simulink model "Chaine_de_conversion_eolienne_25kw"  (R2024a)
settings: Solver=FixedStepAuto  StartTime=0.0  StopTime=10  FixedStep=Ts  RelTol=1e-3
undefined symbols (not defined in the file): A1, A2, A3, A4, A5, A6, C_dc, f, F, G, J, J_PMSG, ki_id_grid, ki_iq_grid, ki_isd, ki_omega, ki_PLL, ki_Q, ki_vdc, kp_id_grid, kp_iq_grid, kp_isd, kp_omega, kp_PLL, kp_Q, kp_vdc, Kt, Lf, Ls, p, Phi_r, R, Rf, rho, Rs, S, Ts, Vdc_ref
libraries: eeGeneralControl x12, slpidlib x8, spsThreePhaseVIMeasurementLib x3, eeTransforms x3, spsCurrentMeasurementLib x3, spsVoltageMeasurementLib x3, spsUniversalBridgeLib x2, spsPWMGenerator2LevelLib x2, powerlib_extras x2, spsRMSLib x2, spsTHDLib x2, spsThreePhaseSeriesRLCBranchLib x1
(part 2 of 2)

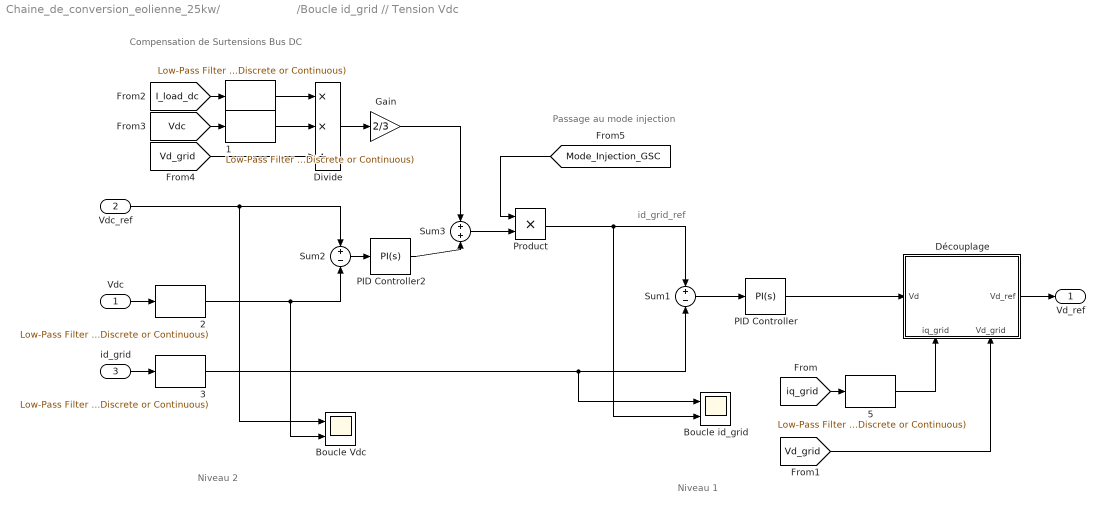
== system Chaine_de_conversion_eolienne_25kw/                       /Boucle id_grid // Tension Vdc ==
  note: Niveau 1
  note: Compensation de Surtensions Bus DC
  note: Passage au mode injection
  note: id_grid_ref
  note: Niveau 2
  Vdc : Inport
  Vdc_ref : Inport  Port=2
  id_grid : Inport  Port=3
  "   " : eeGeneralControl/Low-Pass Filter (Discrete or Continuous)  K=1  T=0.001  B=inf  A=-inf  init_option=Inherited from block input  x0=0  Ts=-1
     {1..3,5} (4 alike) : eeGeneralControl/Low-Pass Filter (Discrete or Continuous)  K=1  T=0.5e-3  B=inf  A=-inf  init_option=Inherited from block input  x0=0  Ts=-1
  Boucle Vdc : Scope  NumInputPorts=2
  "Boucle id_grid   " : Scope  NumInputPorts=2
  Divide : Product  Inputs=**/
  Découplage : Subsystem
      settings: PortSchema="{\"entries\":[{\"content\":{\"sides\":[{\"content\":{\"connectorIds\":[\"In1\"]},\"type\":\"ConnectorPlacement.EquallySpacedRectSide\",\"uuid\":\"7d3af298-2f9f-475a-a651-f5eac2186357\"},{\"content\":{\"connectorIds\":[\"Out1\"],\"side\":\"RIGHT\"},\"type\":\"ConnectorPlacement.EquallySpacedRectSide\",\"uuid\":\"aa22588b-a98c-4a55-adf5-26eaad5d3043\"},{\"content\":{\"side\":\"TOP\"},\"type\":\"ConnectorPlacement.EquallySpacedRectSide\",\"uuid\":\"895af8ff-ad69-460f-8331-727a35d5d5ec\"},{\"content\":{\"connectorIds\":[\"In2\",\"In3\"],\"side\":\"BOTTOM\"},\"type\":\"ConnectorPlacement.EquallySpacedRectSide\",\"uuid\":\"a79db6ec-2ceb-4bca-883f-aa3bf861af08\"}]},\"type\":\"ConnectorPlacement.EquallySpacedConnector\",\"uuid\":\"f85c84fc-5e67-455b-b890-ed27a42cb9c3\"}],\"packageUris\":[\"http://schema.mathworks.com/mf0/Connector/R2020b\"],\"version\":\"1.0\"}"
  Gain : Gain  Gain=2/3
  PID Controller : slpidlib/PID Controller  Controller=PI  Form=Parallel  TimeDomain=Continuous-time  UseExternalTs=off  SampleTime=-1  IntegratorMethod=Forward Euler  FilterMethod=Forward Euler  ControllerParametersSource=internal  P=kp_id_grid  I=ki_id_grid  UseKiTs=off  D=0  UseExternalDerivativeSource=off  N=100  UseFilter=on  TunerSelectOption=Transfer Function Based (PID Tuner App)  InitialConditionSource=internal  InitialConditionForIntegrator=0  InitialConditionForFilter=0  DifferentiatorICPrevScaledInput=0  ExternalReset=none  TrackingMode=off  Kt=1  LimitOutput=off  SatLimitsSource=internal  UpperSaturationLimit=inf  LowerSaturationLimit=-inf  LinearizeAsGain=on  AntiWindupMode=none  Kb=1  LimitIntegrator=off  UpperIntegratorSaturationLimit=inf  LowerIntegratorSaturationLimit=-inf  POutMin=[]  POutMax=[]  IOutMin=[]  IOutMax=[]  DOutMin=[]  DOutMax=[]  NOutMin=[]  NOutMax=[]  SumOutMin=[]  SumOutMax=[]  SaturationOutMin=[]  SaturationOutMax=[]  PParamMin=[]  PParamMax=[]  IParamMin=[]  IParamMax=[]  DParamMin=[]  DParamMax=[]  NParamMin=[]  NParamMax=[]  KbParamMin=[]  KbParamMax=[]  KtParamMin=[]  KtParamMax=[]  KbOutMin=[]  KbOutMax=[]  KtOutMin=[]  KtOutMax=[]  IntegratorOutMin=[]  IntegratorOutMax=[]  FilterOutMin=[]  FilterOutMax=[]  SumI1OutMin=[]  SumI1OutMax=[]  SumI2OutMin=[]  SumI2OutMax=[]  SumI3OutMin=[]  SumI3OutMax=[]  SumI4OutMin=[]  SumI4OutMax=[]  SumDOutMin=[]  SumDOutMax=[]  DifferentiatorOutMin=[]  DifferentiatorOutMax=[]  FilterDiffOutCoefMin=[]  FilterDiffOutCoefMax=[]  ReciprocalOutMin=[]  ReciprocalOutMax=[]  SumDenOutMin=[]  SumDenOutMax=[]  SumNumOutMin=[]  SumNumOutMax=[]  DivideOutMin=[]  DivideOutMax=[]  UdiffTsProdOutMin=[]  UdiffTsProdOutMax=[]  NTsProdOutMin=[]  NTsProdOutMax=[]  UintegralTsProdOutMin=[]  UintegralTsProdOutMax=[]  UngainTsProdOutMin=[]  UngainTsProdOutMax=[]  ClampingZeroOutDataTypeStr=Inherit: Inherit via back propagation  ClampingZeroOutMin=[]  ClampingZeroOutMax=[]  FilterDenConstantOutDataTypeStr=Inherit: Inherit via back propagation  FilterDenConstantOutMin=[]  FilterDenConstantOutMax=[]  PCopyOutDataTypeStr=Inherit: Inherit via back propagation  PCopyOutMin=[]  PCopyOutMax=[]  NCopyOutDataTypeStr=Inherit: Inherit via back propagation  NCopyOutMin=[]  NCopyOutMax=[]  IntegratorContinuousStateAttributes=''  IntegratorStateMustResolveToSignalObject=off  IntegratorRTWStateStorageClass=Auto  FilterContinuousStateAttributes=''  FilterStateMustResolveToSignalObject=off  FilterRTWStateStorageClass=Auto  ParallelPVariant=InternalParameters  IdealPVariant=Disabled  IVariant=InternalParameters  DVariant=Disabled  IntegratorVariant=Continuous  SatVariant=Disabled  AWVariant=Passthrough  PCopyVariant=Disabled  TRVariant=Disabled  FdbkBlocksVariant=Forward  IdealPFdbkVariant=Disabled  SatFdbkVariant=Disabled  DerivativeFilterVariant=Disabled  NVariant=Disabled  NCopyVariant=Disabled_SignalSpec  FilterICVariant=Disabled  IntegratorICVariant=InternalICs  ExternalResetVariant=Disabled  TRSumVariant=Passthrough  SumFdbkVariant=Disabled  SumVariant=Sum_PI  TsampFilterVariant=InternalTs  TsampNgainVariant=Passthrough  TsampIntegralVariant=Disabled_SignalSpec  ExternalSaturationOutDataTypeStr=Inherit: Same as second input  DerivativeSourceVariant=Disabled
  PID Controller2 : slpidlib/PID Controller  Controller=PI  Form=Parallel  TimeDomain=Continuous-time  UseExternalTs=off  SampleTime=-1  IntegratorMethod=Forward Euler  FilterMethod=Forward Euler  ControllerParametersSource=internal  P=kp_vdc  I=ki_vdc  UseKiTs=off  D=0  UseExternalDerivativeSource=off  N=100  UseFilter=on  TunerSelectOption=Transfer Function Based (PID Tuner App)  InitialConditionSource=internal  InitialConditionForIntegrator=0  InitialConditionForFilter=0  DifferentiatorICPrevScaledInput=0  ExternalReset=none  TrackingMode=off  Kt=1  LimitOutput=off  SatLimitsSource=internal  UpperSaturationLimit=inf  LowerSaturationLimit=-inf  LinearizeAsGain=on  AntiWindupMode=none  Kb=1  LimitIntegrator=off  UpperIntegratorSaturationLimit=inf  LowerIntegratorSaturationLimit=-inf  POutMin=[]  POutMax=[]  IOutMin=[]  IOutMax=[]  DOutMin=[]  DOutMax=[]  NOutMin=[]  NOutMax=[]  SumOutMin=[]  SumOutMax=[]  SaturationOutMin=[]  SaturationOutMax=[]  PParamMin=[]  PParamMax=[]  IParamMin=[]  IParamMax=[]  DParamMin=[]  DParamMax=[]  NParamMin=[]  NParamMax=[]  KbParamMin=[]  KbParamMax=[]  KtParamMin=[]  KtParamMax=[]  KbOutMin=[]  KbOutMax=[]  KtOutMin=[]  KtOutMax=[]  IntegratorOutMin=[]  IntegratorOutMax=[]  FilterOutMin=[]  FilterOutMax=[]  SumI1OutMin=[]  SumI1OutMax=[]  SumI2OutMin=[]  SumI2OutMax=[]  SumI3OutMin=[]  SumI3OutMax=[]  SumI4OutMin=[]  SumI4OutMax=[]  SumDOutMin=[]  SumDOutMax=[]  DifferentiatorOutMin=[]  DifferentiatorOutMax=[]  FilterDiffOutCoefMin=[]  FilterDiffOutCoefMax=[]  ReciprocalOutMin=[]  ReciprocalOutMax=[]  SumDenOutMin=[]  SumDenOutMax=[]  SumNumOutMin=[]  SumNumOutMax=[]  DivideOutMin=[]  DivideOutMax=[]  UdiffTsProdOutMin=[]  UdiffTsProdOutMax=[]  NTsProdOutMin=[]  NTsProdOutMax=[]  UintegralTsProdOutMin=[]  UintegralTsProdOutMax=[]  UngainTsProdOutMin=[]  UngainTsProdOutMax=[]  ClampingZeroOutDataTypeStr=Inherit: Inherit via back propagation  ClampingZeroOutMin=[]  ClampingZeroOutMax=[]  FilterDenConstantOutDataTypeStr=Inherit: Inherit via back propagation  FilterDenConstantOutMin=[]  FilterDenConstantOutMax=[]  PCopyOutDataTypeStr=Inherit: Inherit via back propagation  PCopyOutMin=[]  PCopyOutMax=[]  NCopyOutDataTypeStr=Inherit: Inherit via back propagation  NCopyOutMin=[]  NCopyOutMax=[]  IntegratorContinuousStateAttributes=''  IntegratorStateMustResolveToSignalObject=off  IntegratorRTWStateStorageClass=Auto  FilterContinuousStateAttributes=''  FilterStateMustResolveToSignalObject=off  FilterRTWStateStorageClass=Auto  ParallelPVariant=InternalParameters  IdealPVariant=Disabled  IVariant=InternalParameters  DVariant=Disabled  IntegratorVariant=Continuous  SatVariant=Disabled  AWVariant=Passthrough  PCopyVariant=Disabled  TRVariant=Disabled  FdbkBlocksVariant=Forward  IdealPFdbkVariant=Disabled  SatFdbkVariant=Disabled  DerivativeFilterVariant=Disabled  NVariant=Disabled  NCopyVariant=Disabled_SignalSpec  FilterICVariant=Disabled  IntegratorICVariant=InternalICs  ExternalResetVariant=Disabled  TRSumVariant=Passthrough  SumFdbkVariant=Disabled  SumVariant=Sum_PI  TsampFilterVariant=InternalTs  TsampNgainVariant=Passthrough  TsampIntegralVariant=Disabled_SignalSpec  ExternalSaturationOutDataTypeStr=Inherit: Same as second input  DerivativeSourceVariant=Disabled
  Product : Product
  Sum1 : Sum  Inputs=+-
  Sum2 : Sum  Inputs=+-
  Sum3 : Sum
  Vd_ref : Outport
  wires:
  Sum1/1 -> PID Controller/1
  id_grid/1 -> "   3"/1
  Découplage/1(Vd_ref) -> Vd_ref/1
  Sum2/1 -> PID Controller2/1
  Vdc/1 -> "   2"/1
  Vdc_ref/1 -> Boucle Vdc/1, Sum2/1
  Product/1 -> "Boucle id_grid   "/2, Sum1/1
  PID Controller2/1 -> Sum3/2
  PID Controller/1 -> Découplage/1(Vd)
  [iq_grid] -> "   5"/1
  Divide/1 -> Gain/1
  Gain/1 -> Sum3/1
  [Vdc] -> "   1"/1
  [Vd_grid] -> Divide/3
  [I_load_dc] -> "   "/1
  "   "/1 -> Divide/1
  "   1"/1 -> Divide/2
  "   2"/1 -> Boucle Vdc/2, Sum2/2
  "   3"/1 -> Sum1/2, "Boucle id_grid   "/1
  [Vd_grid] -> Découplage/3(Vd_grid)
  "   5"/1 -> Découplage/2(iq_grid)
  Sum3/1 -> Product/2
  [Mode_Injection_GSC] -> Product/1

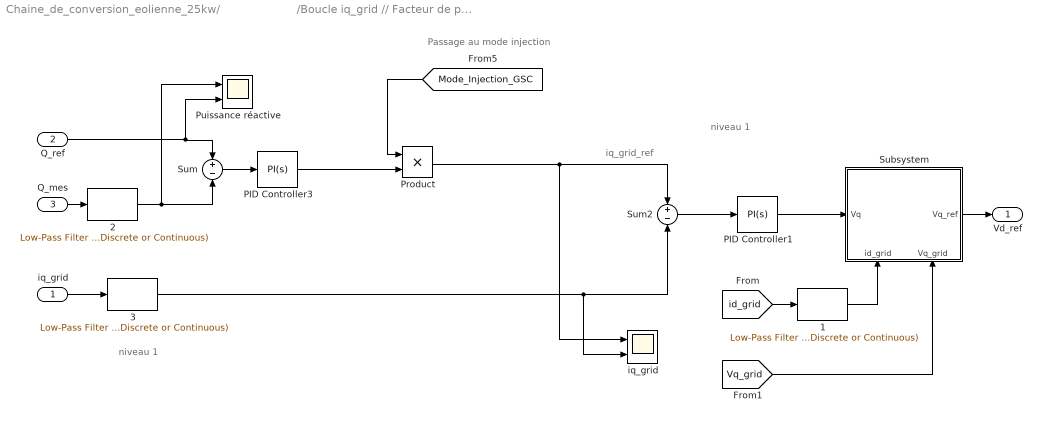
== system Chaine_de_conversion_eolienne_25kw/                       /Boucle iq_grid // Facteur de puissance ==
  note: niveau 1
  note: iq_grid_ref
  note: Passage au mode injection
  note: niveau 1
  iq_grid : Inport
  Q_ref : Inport  Port=2
  Q_mes : Inport  Port=3
  "   1" : eeGeneralControl/Low-Pass Filter (Discrete or Continuous)  K=1  T=0.5e-3  B=inf  A=-inf  init_option=Inherited from block input  x0=0  Ts=-1
  "   2" : eeGeneralControl/Low-Pass Filter (Discrete or Continuous)  K=1  T=0.5e-3  B=inf  A=-inf  init_option=Inherited from block input  x0=0  Ts=-1
  "   3" : eeGeneralControl/Low-Pass Filter (Discrete or Continuous)  K=1  T=0.5e-3  B=inf  A=-inf  init_option=Inherited from block input  x0=0  Ts=-1
  PID Controller1 : slpidlib/PID Controller  Controller=PI  Form=Parallel  TimeDomain=Continuous-time  UseExternalTs=off  SampleTime=-1  IntegratorMethod=Forward Euler  FilterMethod=Forward Euler  ControllerParametersSource=internal  P=kp_iq_grid  I=ki_iq_grid  UseKiTs=off  D=0  UseExternalDerivativeSource=off  N=100  UseFilter=on  TunerSelectOption=Transfer Function Based (PID Tuner App)  InitialConditionSource=internal  InitialConditionForIntegrator=0  InitialConditionForFilter=0  DifferentiatorICPrevScaledInput=0  ExternalReset=none  TrackingMode=off  Kt=1  LimitOutput=off  SatLimitsSource=internal  UpperSaturationLimit=inf  LowerSaturationLimit=-inf  LinearizeAsGain=on  AntiWindupMode=none  Kb=1  LimitIntegrator=off  UpperIntegratorSaturationLimit=inf  LowerIntegratorSaturationLimit=-inf  POutMin=[]  POutMax=[]  IOutMin=[]  IOutMax=[]  DOutMin=[]  DOutMax=[]  NOutMin=[]  NOutMax=[]  SumOutMin=[]  SumOutMax=[]  SaturationOutMin=[]  SaturationOutMax=[]  PParamMin=[]  PParamMax=[]  IParamMin=[]  IParamMax=[]  DParamMin=[]  DParamMax=[]  NParamMin=[]  NParamMax=[]  KbParamMin=[]  KbParamMax=[]  KtParamMin=[]  KtParamMax=[]  KbOutMin=[]  KbOutMax=[]  KtOutMin=[]  KtOutMax=[]  IntegratorOutMin=[]  IntegratorOutMax=[]  FilterOutMin=[]  FilterOutMax=[]  SumI1OutMin=[]  SumI1OutMax=[]  SumI2OutMin=[]  SumI2OutMax=[]  SumI3OutMin=[]  SumI3OutMax=[]  SumI4OutMin=[]  SumI4OutMax=[]  SumDOutMin=[]  SumDOutMax=[]  DifferentiatorOutMin=[]  DifferentiatorOutMax=[]  FilterDiffOutCoefMin=[]  FilterDiffOutCoefMax=[]  ReciprocalOutMin=[]  ReciprocalOutMax=[]  SumDenOutMin=[]  SumDenOutMax=[]  SumNumOutMin=[]  SumNumOutMax=[]  DivideOutMin=[]  DivideOutMax=[]  UdiffTsProdOutMin=[]  UdiffTsProdOutMax=[]  NTsProdOutMin=[]  NTsProdOutMax=[]  UintegralTsProdOutMin=[]  UintegralTsProdOutMax=[]  UngainTsProdOutMin=[]  UngainTsProdOutMax=[]  ClampingZeroOutDataTypeStr=Inherit: Inherit via back propagation  ClampingZeroOutMin=[]  ClampingZeroOutMax=[]  FilterDenConstantOutDataTypeStr=Inherit: Inherit via back propagation  FilterDenConstantOutMin=[]  FilterDenConstantOutMax=[]  PCopyOutDataTypeStr=Inherit: Inherit via back propagation  PCopyOutMin=[]  PCopyOutMax=[]  NCopyOutDataTypeStr=Inherit: Inherit via back propagation  NCopyOutMin=[]  NCopyOutMax=[]  IntegratorContinuousStateAttributes=''  IntegratorStateMustResolveToSignalObject=off  IntegratorRTWStateStorageClass=Auto  FilterContinuousStateAttributes=''  FilterStateMustResolveToSignalObject=off  FilterRTWStateStorageClass=Auto  ParallelPVariant=InternalParameters  IdealPVariant=Disabled  IVariant=InternalParameters  DVariant=Disabled  IntegratorVariant=Continuous  SatVariant=Disabled  AWVariant=Passthrough  PCopyVariant=Disabled  TRVariant=Disabled  FdbkBlocksVariant=Forward  IdealPFdbkVariant=Disabled  SatFdbkVariant=Disabled  DerivativeFilterVariant=Disabled  NVariant=Disabled  NCopyVariant=Disabled_SignalSpec  FilterICVariant=Disabled  IntegratorICVariant=InternalICs  ExternalResetVariant=Disabled  TRSumVariant=Passthrough  SumFdbkVariant=Disabled  SumVariant=Sum_PI  TsampFilterVariant=InternalTs  TsampNgainVariant=Passthrough  TsampIntegralVariant=Disabled_SignalSpec  ExternalSaturationOutDataTypeStr=Inherit: Same as second input  DerivativeSourceVariant=Disabled
  PID Controller3 : slpidlib/PID Controller  Controller=PI  Form=Parallel  TimeDomain=Continuous-time  UseExternalTs=off  SampleTime=-1  IntegratorMethod=Forward Euler  FilterMethod=Forward Euler  ControllerParametersSource=internal  P=kp_Q  I=ki_Q  UseKiTs=off  D=0  UseExternalDerivativeSource=off  N=100  UseFilter=on  TunerSelectOption=Transfer Function Based (PID Tuner App)  InitialConditionSource=internal  InitialConditionForIntegrator=0  InitialConditionForFilter=0  DifferentiatorICPrevScaledInput=0  ExternalReset=none  TrackingMode=off  Kt=1  LimitOutput=off  SatLimitsSource=internal  UpperSaturationLimit=inf  LowerSaturationLimit=-inf  LinearizeAsGain=on  AntiWindupMode=none  Kb=1  LimitIntegrator=off  UpperIntegratorSaturationLimit=inf  LowerIntegratorSaturationLimit=-inf  POutMin=[]  POutMax=[]  IOutMin=[]  IOutMax=[]  DOutMin=[]  DOutMax=[]  NOutMin=[]  NOutMax=[]  SumOutMin=[]  SumOutMax=[]  SaturationOutMin=[]  SaturationOutMax=[]  PParamMin=[]  PParamMax=[]  IParamMin=[]  IParamMax=[]  DParamMin=[]  DParamMax=[]  NParamMin=[]  NParamMax=[]  KbParamMin=[]  KbParamMax=[]  KtParamMin=[]  KtParamMax=[]  KbOutMin=[]  KbOutMax=[]  KtOutMin=[]  KtOutMax=[]  IntegratorOutMin=[]  IntegratorOutMax=[]  FilterOutMin=[]  FilterOutMax=[]  SumI1OutMin=[]  SumI1OutMax=[]  SumI2OutMin=[]  SumI2OutMax=[]  SumI3OutMin=[]  SumI3OutMax=[]  SumI4OutMin=[]  SumI4OutMax=[]  SumDOutMin=[]  SumDOutMax=[]  DifferentiatorOutMin=[]  DifferentiatorOutMax=[]  FilterDiffOutCoefMin=[]  FilterDiffOutCoefMax=[]  ReciprocalOutMin=[]  ReciprocalOutMax=[]  SumDenOutMin=[]  SumDenOutMax=[]  SumNumOutMin=[]  SumNumOutMax=[]  DivideOutMin=[]  DivideOutMax=[]  UdiffTsProdOutMin=[]  UdiffTsProdOutMax=[]  NTsProdOutMin=[]  NTsProdOutMax=[]  UintegralTsProdOutMin=[]  UintegralTsProdOutMax=[]  UngainTsProdOutMin=[]  UngainTsProdOutMax=[]  ClampingZeroOutDataTypeStr=Inherit: Inherit via back propagation  ClampingZeroOutMin=[]  ClampingZeroOutMax=[]  FilterDenConstantOutDataTypeStr=Inherit: Inherit via back propagation  FilterDenConstantOutMin=[]  FilterDenConstantOutMax=[]  PCopyOutDataTypeStr=Inherit: Inherit via back propagation  PCopyOutMin=[]  PCopyOutMax=[]  NCopyOutDataTypeStr=Inherit: Inherit via back propagation  NCopyOutMin=[]  NCopyOutMax=[]  IntegratorContinuousStateAttributes=''  IntegratorStateMustResolveToSignalObject=off  IntegratorRTWStateStorageClass=Auto  FilterContinuousStateAttributes=''  FilterStateMustResolveToSignalObject=off  FilterRTWStateStorageClass=Auto  ParallelPVariant=InternalParameters  IdealPVariant=Disabled  IVariant=InternalParameters  DVariant=Disabled  IntegratorVariant=Continuous  SatVariant=Disabled  AWVariant=Passthrough  PCopyVariant=Disabled  TRVariant=Disabled  FdbkBlocksVariant=Forward  IdealPFdbkVariant=Disabled  SatFdbkVariant=Disabled  DerivativeFilterVariant=Disabled  NVariant=Disabled  NCopyVariant=Disabled_SignalSpec  FilterICVariant=Disabled  IntegratorICVariant=InternalICs  ExternalResetVariant=Disabled  TRSumVariant=Passthrough  SumFdbkVariant=Disabled  SumVariant=Sum_PI  TsampFilterVariant=InternalTs  TsampNgainVariant=Passthrough  TsampIntegralVariant=Disabled_SignalSpec  ExternalSaturationOutDataTypeStr=Inherit: Same as second input  DerivativeSourceVariant=Disabled
  Product : Product
  Puissance réactive : Scope  NumInputPorts=2
  Subsystem : Subsystem
      settings: PortSchema="{\"entries\":[{\"content\":{\"sides\":[{\"content\":{\"connectorIds\":[\"In1\"]},\"type\":\"ConnectorPlacement.EquallySpacedRectSide\",\"uuid\":\"7d3af298-2f9f-475a-a651-f5eac2186357\"},{\"content\":{\"connectorIds\":[\"Out1\"],\"side\":\"RIGHT\"},\"type\":\"ConnectorPlacement.EquallySpacedRectSide\",\"uuid\":\"aa22588b-a98c-4a55-adf5-26eaad5d3043\"},{\"content\":{\"side\":\"TOP\"},\"type\":\"ConnectorPlacement.EquallySpacedRectSide\",\"uuid\":\"895af8ff-ad69-460f-8331-727a35d5d5ec\"},{\"content\":{\"connectorIds\":[\"In2\",\"In3\"],\"side\":\"BOTTOM\"},\"type\":\"ConnectorPlacement.EquallySpacedRectSide\",\"uuid\":\"a79db6ec-2ceb-4bca-883f-aa3bf861af08\"}]},\"type\":\"ConnectorPlacement.EquallySpacedConnector\",\"uuid\":\"f85c84fc-5e67-455b-b890-ed27a42cb9c3\"}],\"packageUris\":[\"http://schema.mathworks.com/mf0/Connector/R2020b\"],\"version\":\"1.0\"}"
  Sum : Sum  Inputs=+-
  Sum2 : Sum  Inputs=+-
  "iq_grid " : Scope  NumInputPorts=2
  Vd_ref : Outport
  wires:
  Sum/1 -> PID Controller3/1
  Sum2/1 -> PID Controller1/1
  iq_grid/1 -> "   3"/1
  Q_mes/1 -> "   2"/1
  Product/1 -> "iq_grid "/1, Sum2/1
  [id_grid] -> "   1"/1
  PID Controller1/1 -> Subsystem/1(Vq)
  Subsystem/1(Vq_ref) -> Vd_ref/1
  [Vq_grid] -> Subsystem/3(Vq_grid)
  "   3"/1 -> Sum2/2, "iq_grid "/2
  Q_ref/1 -> Sum/1, Puissance réactive/2
  "   2"/1 -> Sum/2, Puissance réactive/1
  "   1"/1 -> Subsystem/2(id_grid)
  [Mode_Injection_GSC] -> Product/1
  PID Controller3/1 -> Product/2

== system Chaine_de_conversion_eolienne_25kw/                       /Convertisseur Tension// PWM  ==
  abc_ref : Inport
  Divide3 : Product  Inputs=*/
  PWM Generator (2-Level) : spsPWMGenerator2LevelLib/PWM Generator (2-Level)  ModulatorType=Three-phase bridge (6 pulses)  ModulatorMode=Unsynchronized  Fc=Fc  Pc=90  nF=27  MinMax="[ -1  1 ]"  SamplingTechnique=Natural  ModulatingSignals=off  m=0.8  Freq=60  Phase=0  Ts=Ts  ShowCarrierOutport=off
  Scope : Scope
  Unit Delay1 : UnitDelay  SampleTime=Ts  HasFrameUpgradeWarning=on
  indiceM=33_(1/(fr*33)3 : Constant  Value=(Vdc_ref / 2)
  P1 : Outport
  wires:
  indiceM=33_(1/(fr*33)3/1 -> Divide3/2
  abc_ref/1 -> Divide3/1
  PWM Generator (2-Level)/1 -> P1/1
  Unit Delay1/1 -> PWM Generator (2-Level)/1, Scope/1
  Divide3/1 -> Unit Delay1/1

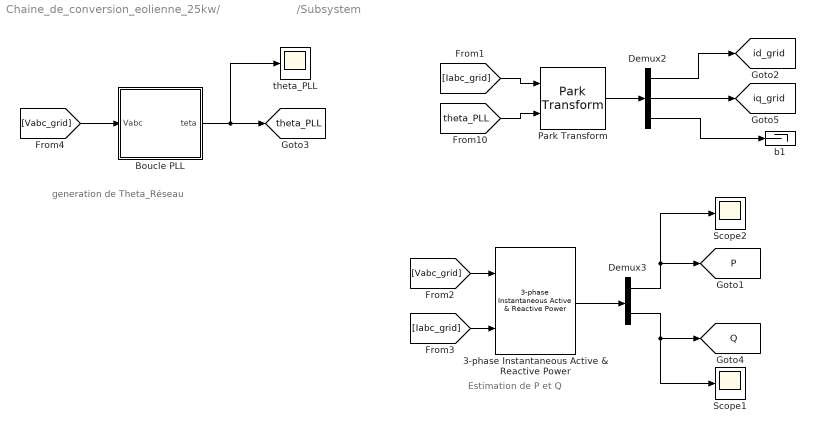
== system Chaine_de_conversion_eolienne_25kw/                       /Subsystem ==
  note: generation de Theta_Réseau
  note: Estimation de P et Q
  3-phase Instantaneous Active & Reactive Power : powerlib_extras/Measurements/3-phase  Instantaneous  Active & Reactive Power
  Boucle PLL : Subsystem
  Demux2 : Demux  Outputs=3
      settings: DisplayOption=none
  Demux3 : Demux  Outputs=2
      settings: DisplayOption=none
  Park Transform : eeTransforms/Park Transform  AxisAlignment=Q-axis  PowerInvariant=off
      settings: LibrarySourceBlock=|
      | ee_sl_lib/Mathematical
      | Transforms/Park Transform
  Scope1 : Scope
  Scope2 : Scope
  b1 : Terminator
  theta_PLL : Scope
  tag scope: P=global, Q=global, id_grid=global, iq_grid=global, theta_PLL=global
  wires:
  [theta_PLL] -> Park Transform/2
  Boucle PLL/1(teta) -> theta_PLL/1, [theta_PLL]
  Demux3/2 -> Scope1/1, [Q]
  Demux2/3 -> b1/1
  3-phase Instantaneous Active & Reactive Power/1 -> Demux3/1
  Park Transform/1 -> Demux2/1
  Demux2/1 -> [id_grid]
  Demux2/2 -> [iq_grid]
  [Iabc_grid] -> Park Transform/1
  [Vabc_grid] -> 3-phase Instantaneous Active & Reactive Power/1
  [Iabc_grid] -> 3-phase Instantaneous Active & Reactive Power/2
  [Vabc_grid] -> Boucle PLL/1(Vabc)
  Demux3/1 -> Scope2/1, [P]

== system Chaine_de_conversion_eolienne_25kw/                 /Boucle id // découplage vq/Découplage Axe d ==
  note: Vd_ref = Vd_PI - (ω_e × Ls × isq)
  vd : Inport
  Iq : Inport  Port=2
  Wm : Inport  Port=3
  Product3 : Product  SaturateOnIntegerOverflow=on  OutDataTypeStr=Inherit: Same as first input
  Sum2 : Sum  Inputs=+-  SaturateOnIntegerOverflow=on
  u2 : Gain  Gain=Ls*p  SaturateOnIntegerOverflow=on  OutDataTypeStr=Inherit: Same as input  ParamDataTypeStr=Inherit: Same as input
  Vdref : Outport
  wires:
  Sum2/1 -> Vdref/1
  Wm/1 -> Product3/2
  Iq/1 -> Product3/1
  Product3/1 -> u2/1
  vd/1 -> Sum2/1
  u2/1 -> Sum2/2

== system Chaine_de_conversion_eolienne_25kw/                 /Boucle iq // découplage vq/Découplage ==
  note: Vq_ref = Vq_PI + (ω_e × Ls × isd) + (ω_e × Φ_r)
  vq : Inport
  Id : Inport  Port=2
  Wm : Inport  Port=3
  Product3 : Product  SaturateOnIntegerOverflow=on  OutDataTypeStr=Inherit: Same as first input
  Sum2 : Sum  Inputs=+++  SaturateOnIntegerOverflow=on
  u1 : Gain  Gain=p*Phi_r  SaturateOnIntegerOverflow=on  OutDataTypeStr=Inherit: Same as input  ParamDataTypeStr=Inherit: Same as input
  u2 : Gain  Gain=p*Ls  SaturateOnIntegerOverflow=on  OutDataTypeStr=Inherit: Same as input  ParamDataTypeStr=Inherit: Same as input
  Vqref : Outport
  wires:
  vq/1 -> Sum2/1
  Product3/1 -> u2/1
  Id/1 -> Product3/1
  Wm/1 -> u1/1, Product3/2
  Sum2/1 -> Vqref/1
  u2/1 -> Sum2/2
  u1/1 -> Sum2/3

== system Chaine_de_conversion_eolienne_25kw/                       /Boucle id_grid // Tension Vdc/Découplage ==
  Vd : Inport
  iq_grid : Inport  Port=2
  Vd_grid : Inport  Port=3
  Gain : Gain  Gain=-2*pi*f*Lf
  Scope : Scope
  Sum : Sum  Inputs=+++
  Vd_ref : Outport
  wires:
  iq_grid/1 -> Gain/1
  Vd/1 -> Sum/2
  Gain/1 -> Sum/3
  Sum/1 -> Scope/1, Vd_ref/1
  Vd_grid/1 -> Sum/1

== system Chaine_de_conversion_eolienne_25kw/                       /Boucle iq_grid // Facteur de puissance/Subsystem ==
  Vq : Inport
  id_grid : Inport  Port=2
  Vq_grid : Inport  Port=3
  Gain : Gain  Gain=2*pi*f*Lf
  Scope : Scope
  Sum : Sum  Inputs=+++
  Vq_ref : Outport
  wires:
  id_grid/1 -> Gain/1
  Sum/1 -> Scope/1, Vq_ref/1
  Vq_grid/1 -> Sum/1
  Vq/1 -> Sum/2
  Gain/1 -> Sum/3

== system Chaine_de_conversion_eolienne_25kw/                       /Subsystem/Boucle PLL ==
  Vabc : Inport
  Constant1 : Constant  Value=0
  Constant2 : Constant  Value=2*pi*50
  Demux : Demux  Outputs=3
  Integrator2 : Integrator
  Mux : Mux  Inputs=2
  Sum1 : Sum  SaturateOnIntegerOverflow=on
  Sum3 : Sum  Inputs=+-  SaturateOnIntegerOverflow=on
  Trigonometric Function : Trigonometry
  Trigonometric Function1 : Trigonometry  Operator=cos
  abc_to_dq0 Transformation1 : powerlib_extras/Measurements/abc_to_dq0 Transformation
  b1 : Terminator
  pll : Subsystem
  teta : Outport
  tag scope: Vd_grid=global, Vq_grid=global
  wires:
  Demux/1 -> [Vd_grid]
  Mux/1 -> abc_to_dq0 Transformation1/2
  Trigonometric Function1/1 -> Mux/2
  Trigonometric Function/1 -> Mux/1
  abc_to_dq0 Transformation1/1 -> Demux/1
  Integrator2/1 -> Trigonometric Function/1, Trigonometric Function1/1, teta/1
  Sum3/1 -> pll/1(Id/idref)
  pll/1(vd) -> Sum1/2
  Constant2/1 -> Sum1/1
  Sum1/1 -> Integrator2/1
  Constant1/1 -> Sum3/1
  Vabc/1 -> abc_to_dq0 Transformation1/1
  Demux/2 -> Sum3/2, [Vq_grid]
  Demux/3 -> b1/1

== system Chaine_de_conversion_eolienne_25kw/                       /Subsystem/Boucle PLL/pll ==
  Id/idref : Inport
  Add : Sum
  Integrator3 : Integrator
  Ki-V_bd_ref : Gain  Gain=ki_PLL  SaturateOnIntegerOverflow=on  OutDataTypeStr=Inherit: Same as input  ParamDataTypeStr=Inherit: Same as input
  Kp-V_bd_ref1 : Gain  Gain=kp_PLL  SaturateOnIntegerOverflow=on  OutDataTypeStr=Inherit: Same as input  ParamDataTypeStr=Inherit: Same as input
  PID Controller : slpidlib/PID Controller  Controller=PID  Form=Parallel  TimeDomain=Continuous-time  UseExternalTs=off  SampleTime=-1  IntegratorMethod=Forward Euler  FilterMethod=Forward Euler  ControllerParametersSource=internal  P=kp_PLL  I=ki_PLL  UseKiTs=off  D=0  UseExternalDerivativeSource=off  N=100  UseFilter=on  TunerSelectOption=Transfer Function Based (PID Tuner App)  InitialConditionSource=internal  InitialConditionForIntegrator=0  InitialConditionForFilter=0  DifferentiatorICPrevScaledInput=0  ExternalReset=none  TrackingMode=off  Kt=1  LimitOutput=off  SatLimitsSource=internal  UpperSaturationLimit=inf  LowerSaturationLimit=-inf  LinearizeAsGain=on  AntiWindupMode=none  Kb=1  LimitIntegrator=off  UpperIntegratorSaturationLimit=inf  LowerIntegratorSaturationLimit=-inf  POutMin=[]  POutMax=[]  IOutMin=[]  IOutMax=[]  DOutMin=[]  DOutMax=[]  NOutMin=[]  NOutMax=[]  SumOutMin=[]  SumOutMax=[]  SaturationOutMin=[]  SaturationOutMax=[]  PParamMin=[]  PParamMax=[]  IParamMin=[]  IParamMax=[]  DParamMin=[]  DParamMax=[]  NParamMin=[]  NParamMax=[]  KbParamMin=[]  KbParamMax=[]  KtParamMin=[]  KtParamMax=[]  KbOutMin=[]  KbOutMax=[]  KtOutMin=[]  KtOutMax=[]  IntegratorOutMin=[]  IntegratorOutMax=[]  FilterOutMin=[]  FilterOutMax=[]  SumI1OutMin=[]  SumI1OutMax=[]  SumI2OutMin=[]  SumI2OutMax=[]  SumI3OutMin=[]  SumI3OutMax=[]  SumI4OutMin=[]  SumI4OutMax=[]  SumDOutMin=[]  SumDOutMax=[]  DifferentiatorOutMin=[]  DifferentiatorOutMax=[]  FilterDiffOutCoefMin=[]  FilterDiffOutCoefMax=[]  ReciprocalOutMin=[]  ReciprocalOutMax=[]  SumDenOutMin=[]  SumDenOutMax=[]  SumNumOutMin=[]  SumNumOutMax=[]  DivideOutMin=[]  DivideOutMax=[]  UdiffTsProdOutMin=[]  UdiffTsProdOutMax=[]  NTsProdOutMin=[]  NTsProdOutMax=[]  UintegralTsProdOutMin=[]  UintegralTsProdOutMax=[]  UngainTsProdOutMin=[]  UngainTsProdOutMax=[]  ClampingZeroOutDataTypeStr=Inherit: Inherit via back propagation  ClampingZeroOutMin=[]  ClampingZeroOutMax=[]  FilterDenConstantOutDataTypeStr=Inherit: Inherit via back propagation  FilterDenConstantOutMin=[]  FilterDenConstantOutMax=[]  PCopyOutDataTypeStr=Inherit: Inherit via back propagation  PCopyOutMin=[]  PCopyOutMax=[]  NCopyOutDataTypeStr=Inherit: Inherit via back propagation  NCopyOutMin=[]  NCopyOutMax=[]  IntegratorContinuousStateAttributes=''  IntegratorStateMustResolveToSignalObject=off  IntegratorRTWStateStorageClass=Auto  FilterContinuousStateAttributes=''  FilterStateMustResolveToSignalObject=off  FilterRTWStateStorageClass=Auto  ParallelPVariant=InternalParameters  IdealPVariant=Disabled  IVariant=InternalParameters  DVariant=InternalParameters  IntegratorVariant=Continuous  SatVariant=Disabled  AWVariant=Passthrough  PCopyVariant=Disabled  TRVariant=Disabled  FdbkBlocksVariant=Forward  IdealPFdbkVariant=Disabled  SatFdbkVariant=Disabled  DerivativeFilterVariant=ContFilter  NVariant=InternalParameters  NCopyVariant=Disabled  FilterICVariant=InternalICsFilter  IntegratorICVariant=InternalICs  ExternalResetVariant=Disabled  TRSumVariant=Passthrough  SumFdbkVariant=Disabled  SumVariant=Sum_PID  TsampFilterVariant=InternalTs  TsampNgainVariant=Passthrough  TsampIntegralVariant=Disabled_SignalSpec  ExternalSaturationOutDataTypeStr=Inherit: Same as second input  DerivativeSourceVariant=ErrorSignal
  vd : Outport
  wires:
  Integrator3/1 -> Add/2
  Ki-V_bd_ref/1 -> Integrator3/1
  Kp-V_bd_ref1/1 -> Add/1
  Id/idref/1 -> PID Controller/1
  PID Controller/1 -> vd/1

== matlab function Chaine_de_conversion_eolienne_25kw/   /Escalier ==
  data: t input; signal output
function signal = generate_step_signal(t)
    % Génère un signal qui varie par paliers constants sur 20 secondes
    % Input : vecteur temps t (en secondes)
    % Output : signal avec des valeurs constantes par segment
    
    signal = zeros(size(t));  % Initialisation du signal
    
    % Définition des intervalles de temps (en secondes) et des valeurs constantes
    segments = [
        0,  4,  12;   % De 0 à 4 sec : valeur = 2.5
        4,  8,  16;   % De 4 à 8 sec : valeur = 1.0
        8,  12, 8;   % De 8 à 12 sec : valeur = 4.0
        12, 16, 14;   % De 12 à 16 sec : valeur = 3.2
        16, 20, 18;   % De 16 à 20 sec : valeur = 0.5
    ];
    
    % Génération du signal par morceaux
    for i = 1:size(segments, 1)
        start_time = segments(i, 1);
        end_time = segments(i, 2);
        value = segments(i, 3);
        
        mask = (t >= start_time) & (t < end_time);
        signal(mask) = value;
    end
    
    % Gestion de la dernière valeur (t = 20)
    signal(t == 20) = segments(end, 3);
end

== matlab function Chaine_de_conversion_eolienne_25kw/Subsystem2/MATLAB Function ==
  data: t input; V_vent input; T_startup output; Omega_ref_init output; Starter_Off output; Omega_mes input; P_cible input; Omega_cible input
function [T_startup, Omega_ref_init, Starter_Off] = Demarreur(t, V_vent, Omega_mes, P_cible, Omega_cible)

    persistent startup_done
    
    if isempty(startup_done)
        startup_done = 0;
    end
      

    T_25kW = P_cible / Omega_cible; 
    
    T_startup = T_25kW;
    Omega_ref_init = Omega_cible;

    
    Seuil_Vitesse_Haute = Omega_cible*0.99;


    if (Omega_mes >= Seuil_Vitesse_Haute) && (V_vent > 5) && (t >=2)
        startup_done = 1; 
        T_startup = 0;
    end
    Starter_Off = startup_done;
end

== matlab function Chaine_de_conversion_eolienne_25kw/   /MATLAB Function3 ==
  data: t input; V_wind output
function V_wind = Wind_Profile(t)
%#codegen
% Profil de vent à rampes avec valeur moyenne = 12 m/s

time_points  = [0.0, 2.0, 5.0, 7.5, 10.0, 15.0, 20.0];
speed_points = [10.3, 11.87, 8, 9, 13, 9, 10];

if t < time_points(1)
    V_wind = speed_points(1);
    return;
end

if t > time_points(end)
    V_wind = speed_points(end);
    return;
end

V_wind = interp1(time_points, speed_points, t, 'linear');

end

== matlab function Chaine_de_conversion_eolienne_25kw/   /MATLAB Function1 ==
  data: t input; V_wind output
function V_wind = Wind_Profile(t)
    % Fonction de profil de vent avec contraintes spécifiques
    % Moyenne = 12, Max = 20, Min = 5
    
    % Points temporels
    time_points = [0.0, 2.0, 5.0, 7.5, 10.0, 15.0, 20.0];
    
    % Nouvelles valeurs ajustées pour respecter les contraintes
    % Calculées pour avoir: moyenne=12, min=5, max=20
    speed_points = [8.5, 12.5, 20, 16.0, 10.5, 5.0, 10.5];
    
    % Gestion des limites temporelles (nécessaire pour Code Generation)
    if t <= time_points(1)
        V_wind = speed_points(1);
    elseif t >= time_points(end)
        V_wind = speed_points(end);
    else
        % Interpolation linéaire
        % Pour la génération de code, utiliser une implémentation manuelle
        V_wind = linear_interp(time_points, speed_points, t);
    end
end

function y = linear_interp(x_vec, y_vec, x)
    % Interpolation linéaire manuelle pour la génération de code
    n = length(x_vec);
    
    % Trouver l'intervalle
    for i = 1:n-1
        if x >= x_vec(i) && x <= x_vec(i+1)
            % Interpolation linéaire
            dx = x_vec(i+1) - x_vec(i);
            if abs(dx) < eps
                y = y_vec(i);
            else
                t = (x - x_vec(i)) / dx;
                y = y_vec(i) + t * (y_vec(i+1) - y_vec(i));
            end
            return;
        end
    end
    
    % Si on arrive ici (ne devrait pas arriver avec les vérifications ci-dessus)
    y = y_vec(end);
end

== matlab function Chaine_de_conversion_eolienne_25kw/      /MATLAB Function2 ==
  data: P_mes input; Omega_ref output; P_betz input; Omega_Start input; Activation input
function Omega_ref = MPPT_Adaptive_PO (P_mes, P_betz,Omega_Start, Activation)
%#codegen
persistent P_prev Omega_ref_prev direction initialized counter;

% --- PARAMÈTRES ---
Omega_min = Omega_Start;
Omega_max = 350;
Eff_est   = 1;

% --- Initialisation ---
if isempty(initialized)
    P_prev = 0;
    Omega_ref_prev = Omega_Start; 
    direction = 1; 
    counter = 0;
    initialized = true;
end

% --- 1. GESTION DU DÉMARRAGE ---
if Activation == 0
    Omega_ref = Omega_Start;
    Omega_ref_prev = Omega_Start; 
    P_prev = P_mes;
    return;
end

% --- 2. TEMPORISATION ---
if counter < 50
    counter = counter + 1;
    Omega_ref = Omega_ref_prev;
    return;
end
counter = 0;

% --- 3. CALCUL DU PAS VARIABLE (MODIFIÉ POUR RAPIDITÉ) ---
P_target = P_betz * Eff_est;
Erreur_P = abs(P_target - P_mes); 

if Erreur_P > 1500
    % Grand écart : Réaction très forte
    Step_Size = 8; 
elseif Erreur_P > 500
    % Écart moyen (Cas t=2s) : Vitesse triplée (passé de 1 à 3)
    Step_Size = 3;  
elseif Erreur_P < 100
    % Zone morte (Stabilisation)
    Step_Size = 0; 
else
    % Ajustement fin
    Step_Size = 0.4; 
end

% --- 4. LOGIQUE P&O STANDARD ---
delta_P = P_mes - P_prev;

% Inversion de direction si la puissance chute
if delta_P < -50
    direction = -direction; 
end

% --- 5. CALCUL FINAL ---
Omega_ref = Omega_ref_prev + (direction * Step_Size);
Omega_ref = max(Omega_min, min(Omega_ref, Omega_max));

% Mises à jour
P_prev = P_mes;
Omega_ref_prev = Omega_ref;

end

== matlab function Chaine_de_conversion_eolienne_25kw/      /MATLAB Function3 ==
  data: V_vent input; P_aero_ref output
function P_aero_ref = Estimateur_Paero(V_vent)
%#codegen
% ESTIMATEUR_PAERO
% Calcule la puissance aérodynamique maximale théorique (P_aero)
% basée sur le Cp_max identifié.

% --- Paramètres Physiques ---
R = 3.96;             % Rayon pale (m)
rho = 1.225;          % Densité air (kg/m^3)
Cp_max = 0.48;        % Coefficient de puissance max (donnée)

% --- Calcul du Gain Optimal (K_opt) ---
% S = Surface balayée (m^2)
S = pi * R^2;

% K_opt = 0.5 * rho * S * Cp_max
% Avec les valeurs : 0.5 * 1.225 * 49.265 * 0.48 ≈ 14.48
K_opt = 0.5 * rho * S * Cp_max;

% --- Calcul de la Puissance Aérodynamique ---
% P = K_opt * V^3
P_aero_ref = K_opt * (V_vent^3);

end

== matlab function Chaine_de_conversion_eolienne_25kw/   /MATLAB Function4 ==
  data: t input; V_wind output
function V_wind = Wind_Profile(t)
%#codegen
% Profil de vent à rampes avec valeur moyenne = 12 m/s

time_points  = [2, 4, 6, 8, 10, 12, 14, 16, 18, 20];
speed_points = [5, 8, 12, 10, 13, 7, 10, 16, 15, 12 ];

if t < time_points(1)
    V_wind = speed_points(1);
    return;
end

if t > time_points(end)
    V_wind = speed_points(end);
    return;
end

V_wind = interp1(time_points, speed_points, t, 'linear');

end
